simulink model "AutoPilot"  (R2013a)
settings: Solver=ode45  StartTime=0.0  StopTime=10.0  RelTol=1e-3
libraries: simulink x10
settings Model: Creator=falk  LastModifiedBy=falk

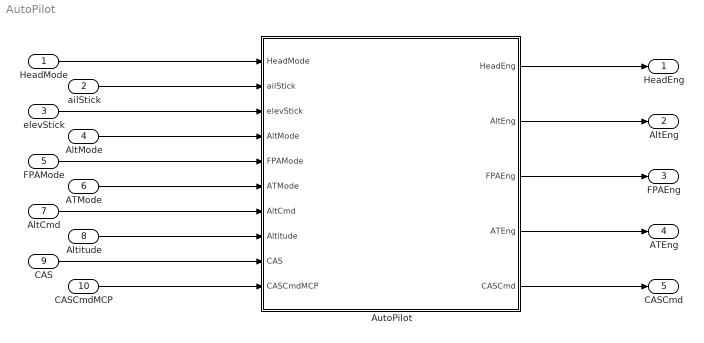
== system AutoPilot ==
  HeadMode : Inport
  ailStick : Inport  Port=2
  elevStick : Inport  Port=3
  AltMode : Inport  Port=4
  FPAMode : Inport  Port=5
  ATMode : Inport  Port=6
  AltCmd : Inport  Port=7
  Altitude : Inport  Port=8
  CAS : Inport  Port=9
  CASCmdMCP : Inport  Port=10
  AutoPilot : Subsystem
  HeadEng : Outport
  AltEng : Outport  Port=2
  FPAEng : Outport  Port=3
  ATEng : Outport  Port=4
  CASCmd : Outport  Port=5
  wires:
  HeadMode/1 -> AutoPilot/1(HeadMode)
  ailStick/1 -> AutoPilot/2(ailStick)
  elevStick/1 -> AutoPilot/3(elevStick)
  AltMode/1 -> AutoPilot/4(AltMode)
  FPAMode/1 -> AutoPilot/5(FPAMode)
  ATMode/1 -> AutoPilot/6(ATMode)
  AltCmd/1 -> AutoPilot/7(AltCmd)
  Altitude/1 -> AutoPilot/8(Altitude)
  CAS/1 -> AutoPilot/9(CAS)
  CASCmdMCP/1 -> AutoPilot/10(CASCmdMCP)
  AutoPilot/1(HeadEng) -> HeadEng/1
  AutoPilot/2(AltEng) -> AltEng/1
  AutoPilot/3(FPAEng) -> FPAEng/1
  AutoPilot/4(ATEng) -> ATEng/1
  AutoPilot/5(CASCmd) -> CASCmd/1

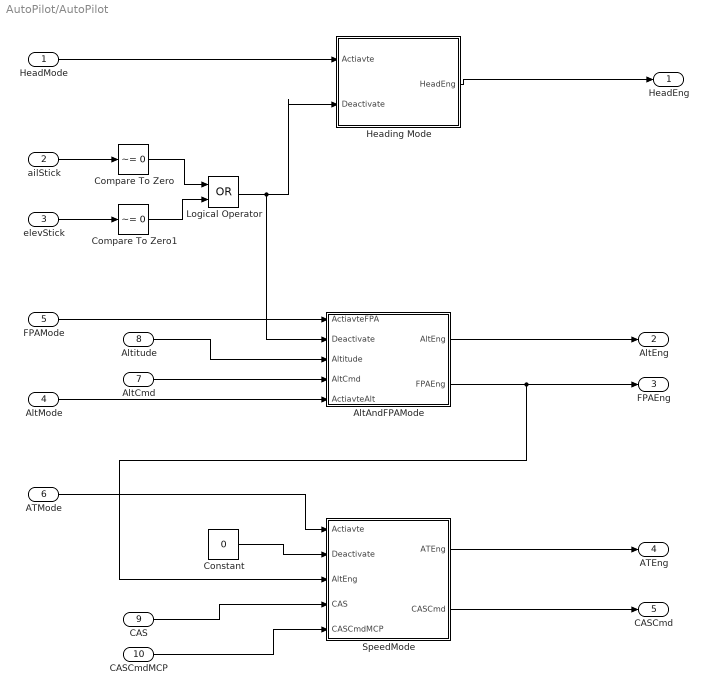
== system AutoPilot/AutoPilot ==
  HeadMode : Inport
  ailStick : Inport  Port=2
  elevStick : Inport  Port=3
  AltMode : Inport  Port=4
  FPAMode : Inport  Port=5
  ATMode : Inport  Port=6
  AltCmd : Inport  Port=7
  Altitude : Inport  Port=8
  CAS : Inport  Port=9
  CASCmdMCP : Inport  Port=10
  AltAndFPAMode : Subsystem
  Compare To Zero : simulink/Logic and Bit Operations/Compare To Zero  relop=~=  OutDataTypeStr=boolean
  Compare To Zero1 : simulink/Logic and Bit Operations/Compare To Zero  relop=~=  OutDataTypeStr=boolean
  Constant : Constant  Value=0
  Heading Mode : Subsystem
  Logical Operator : Logic  Operator=OR  AllPortsSameDT=off  OutDataTypeStr=boolean
  SpeedMode : Subsystem
  HeadEng : Outport
  AltEng : Outport  Port=2
  FPAEng : Outport  Port=3
  ATEng : Outport  Port=4
  CASCmd : Outport  Port=5
  wires:
  SpeedMode/1(ATEng) -> ATEng/1
  ailStick/1 -> Compare To Zero/1
  Constant/1 -> SpeedMode/2(Deactivate)
  AltAndFPAMode/2(FPAEng) -> FPAEng/1, SpeedMode/3(AltEng)
  AltAndFPAMode/1(AltEng) -> AltEng/1
  Heading Mode/1(HeadEng) -> HeadEng/1
  HeadMode/1 -> Heading Mode/1(Actiavte)
  Compare To Zero1/1 -> Logical Operator/2
  Compare To Zero/1 -> Logical Operator/1
  elevStick/1 -> Compare To Zero1/1
  ATMode/1 -> SpeedMode/1(Actiavte)
  FPAMode/1 -> AltAndFPAMode/1(ActiavteFPA)
  Altitude/1 -> AltAndFPAMode/3(Altitude)
  AltMode/1 -> AltAndFPAMode/5(ActiavteAlt)
  Logical Operator/1 -> AltAndFPAMode/2(Deactivate), Heading Mode/2(Deactivate)
  CASCmdMCP/1 -> SpeedMode/5(CASCmdMCP)
  AltCmd/1 -> AltAndFPAMode/4(AltCmd)
  SpeedMode/2(CASCmd) -> CASCmd/1
  CAS/1 -> SpeedMode/4(CAS)

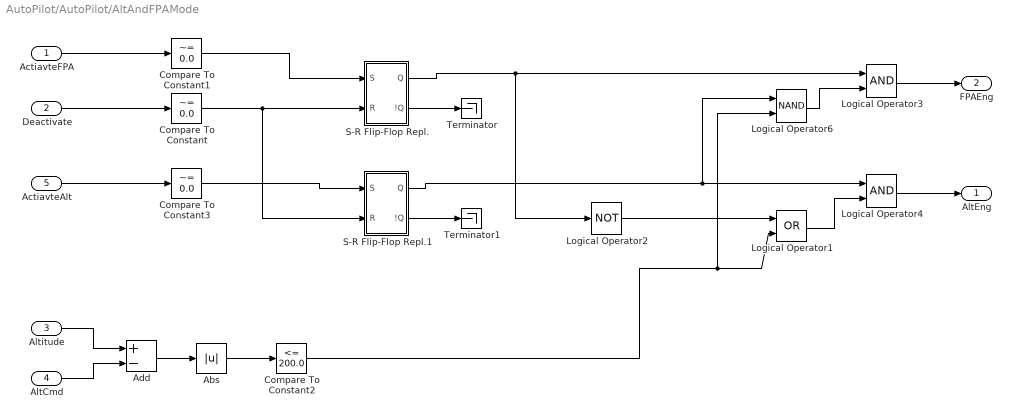
== system AutoPilot/AutoPilot/AltAndFPAMode ==
  ActiavteFPA : Inport
  Deactivate : Inport  Port=2
  Altitude : Inport  Port=3
  AltCmd : Inport  Port=4
  ActiavteAlt : Inport  Port=5
  Abs : Abs
  Add : Sum  Inputs=+-
  Compare To Constant : simulink/Logic and Bit Operations/Compare To Constant  relop=~=  const=0.0  OutDataTypeStr=boolean
  Compare To Constant1 : simulink/Logic and Bit Operations/Compare To Constant  relop=~=  const=0.0  OutDataTypeStr=boolean
  Compare To Constant2 : simulink/Logic and Bit Operations/Compare To Constant  relop=<=  const=200.0  OutDataTypeStr=boolean
  Compare To Constant3 : simulink/Logic and Bit Operations/Compare To Constant  relop=~=  const=0.0  OutDataTypeStr=boolean
  Logical Operator1 : Logic  Operator=OR  AllPortsSameDT=off  OutDataTypeStr=boolean
  Logical Operator2 : Logic  Operator=NOT  AllPortsSameDT=off  OutDataTypeStr=boolean
  Logical Operator3 : Logic  AllPortsSameDT=off  OutDataTypeStr=boolean
  Logical Operator4 : Logic  AllPortsSameDT=off  OutDataTypeStr=boolean
  Logical Operator6 : Logic  Operator=NAND  AllPortsSameDT=off  OutDataTypeStr=boolean
  S-R Flip-Flop Repl. : Subsystem
  S-R Flip-Flop Repl.1 : Subsystem
  Terminator : Terminator
  Terminator1 : Terminator
  AltEng : Outport
  FPAEng : Outport  Port=2
  wires:
  S-R Flip-Flop Repl./2(!Q) -> Terminator/1
  ActiavteFPA/1 -> Compare To Constant1/1
  S-R Flip-Flop Repl./1(Q) -> Logical Operator3/1, Logical Operator2/1
  Deactivate/1 -> Compare To Constant/1
  Compare To Constant1/1 -> S-R Flip-Flop Repl./1(S)
  S-R Flip-Flop Repl.1/2(!Q) -> Terminator1/1
  S-R Flip-Flop Repl.1/1(Q) -> Logical Operator6/1, Logical Operator4/1
  Compare To Constant3/1 -> S-R Flip-Flop Repl.1/1(S)
  Compare To Constant/1 -> S-R Flip-Flop Repl.1/2(R), S-R Flip-Flop Repl./2(R)
  ActiavteAlt/1 -> Compare To Constant3/1
  Altitude/1 -> Add/1
  AltCmd/1 -> Add/2
  Add/1 -> Abs/1
  Abs/1 -> Compare To Constant2/1
  Logical Operator3/1 -> FPAEng/1
  Logical Operator2/1 -> Logical Operator1/1
  Logical Operator4/1 -> AltEng/1
  Compare To Constant2/1 -> Logical Operator6/2, Logical Operator1/2
  Logical Operator1/1 -> Logical Operator4/2
  Logical Operator6/1 -> Logical Operator3/2

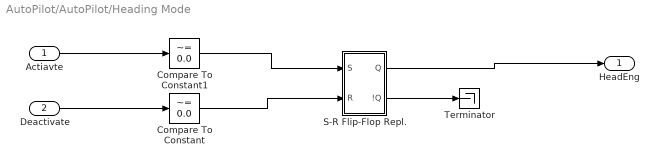
== system AutoPilot/AutoPilot/Heading Mode ==
  Actiavte : Inport
  Deactivate : Inport  Port=2
  Compare To Constant : simulink/Logic and Bit Operations/Compare To Constant  relop=~=  const=0.0  OutDataTypeStr=boolean
  Compare To Constant1 : simulink/Logic and Bit Operations/Compare To Constant  relop=~=  const=0.0  OutDataTypeStr=boolean
  S-R Flip-Flop Repl. : Subsystem
  Terminator : Terminator
  HeadEng : Outport
  wires:
  S-R Flip-Flop Repl./2(!Q) -> Terminator/1
  Actiavte/1 -> Compare To Constant1/1
  S-R Flip-Flop Repl./1(Q) -> HeadEng/1
  Deactivate/1 -> Compare To Constant/1
  Compare To Constant1/1 -> S-R Flip-Flop Repl./1(S)
  Compare To Constant/1 -> S-R Flip-Flop Repl./2(R)

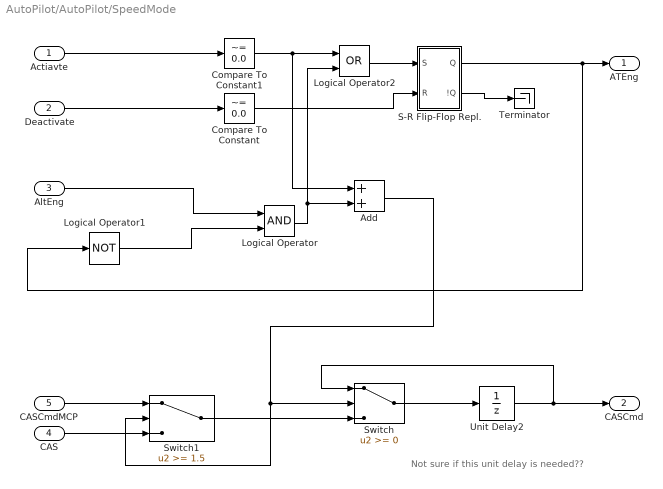
== system AutoPilot/AutoPilot/SpeedMode ==
  note: Not sure if this unit delay is needed??
  Actiavte : Inport
  Deactivate : Inport  Port=2
  AltEng : Inport  Port=3
  CAS : Inport  Port=4
  CASCmdMCP : Inport  Port=5
  Add : Sum
  Compare To Constant : simulink/Logic and Bit Operations/Compare To Constant  relop=~=  const=0.0  OutDataTypeStr=boolean
  Compare To Constant1 : simulink/Logic and Bit Operations/Compare To Constant  relop=~=  const=0.0  OutDataTypeStr=boolean
  Logical Operator : Logic  AllPortsSameDT=off  OutDataTypeStr=boolean
  Logical Operator1 : Logic  Operator=NOT  AllPortsSameDT=off  OutDataTypeStr=boolean
  Logical Operator2 : Logic  Operator=OR  AllPortsSameDT=off  OutDataTypeStr=boolean
  S-R Flip-Flop Repl. : Subsystem
  Switch : Switch
  Switch1 : Switch  Threshold=1.5
  Terminator : Terminator
  Unit Delay2 : UnitDelay  SampleTime=-1
  ATEng : Outport
  CASCmd : Outport  Port=2
  wires:
  S-R Flip-Flop Repl./2(!Q) -> Terminator/1
  Actiavte/1 -> Compare To Constant1/1
  S-R Flip-Flop Repl./1(Q) -> Logical Operator1/1, ATEng/1
  Deactivate/1 -> Compare To Constant/1
  Compare To Constant/1 -> S-R Flip-Flop Repl./2(R)
  AltEng/1 -> Logical Operator/1
  Logical Operator1/1 -> Logical Operator/2
  Logical Operator2/1 -> S-R Flip-Flop Repl./1(S)
  Logical Operator/1 -> Add/2, Logical Operator2/2
  CAS/1 -> Switch1/3
  CASCmdMCP/1 -> Switch1/1
  Compare To Constant1/1 -> Add/1, Logical Operator2/1
  Add/1 -> Switch1/2, Switch/2
  Switch1/1 -> Switch/3
  Switch/1 -> Unit Delay2/1
  Unit Delay2/1 -> Switch/1, CASCmd/1

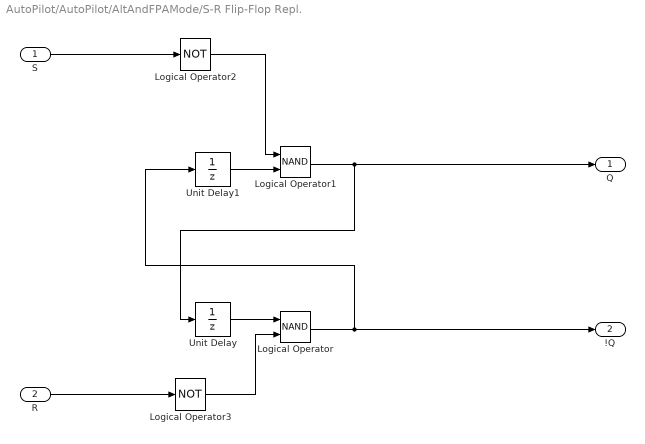
== system AutoPilot/AutoPilot/AltAndFPAMode/S-R Flip-Flop Repl. ==
  S : Inport
  R : Inport  Port=2
  Logical Operator : Logic  Operator=NAND  AllPortsSameDT=off  OutDataTypeStr=boolean
  Logical Operator1 : Logic  Operator=NAND  AllPortsSameDT=off  OutDataTypeStr=boolean
  Logical Operator2 : Logic  Operator=NOT  AllPortsSameDT=off  OutDataTypeStr=boolean
  Logical Operator3 : Logic  Operator=NOT  AllPortsSameDT=off  OutDataTypeStr=boolean
  Unit Delay : UnitDelay  SampleTime=-1
  Unit Delay1 : UnitDelay  InitialCondition=1  SampleTime=-1
  Q : Outport
  !Q : Outport  Port=2
  wires:
  Logical Operator/1 -> Unit Delay1/1, !Q/1
  Logical Operator1/1 -> Unit Delay/1, Q/1
  Unit Delay/1 -> Logical Operator/1
  Unit Delay1/1 -> Logical Operator1/2
  Logical Operator2/1 -> Logical Operator1/1
  Logical Operator3/1 -> Logical Operator/2
  R/1 -> Logical Operator3/1
  S/1 -> Logical Operator2/1

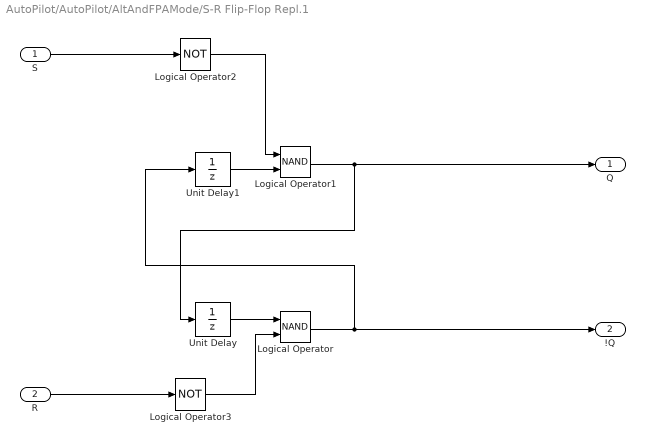
== system AutoPilot/AutoPilot/AltAndFPAMode/S-R Flip-Flop Repl.1 ==
  S : Inport
  R : Inport  Port=2
  Logical Operator : Logic  Operator=NAND  AllPortsSameDT=off  OutDataTypeStr=boolean
  Logical Operator1 : Logic  Operator=NAND  AllPortsSameDT=off  OutDataTypeStr=boolean
  Logical Operator2 : Logic  Operator=NOT  AllPortsSameDT=off  OutDataTypeStr=boolean
  Logical Operator3 : Logic  Operator=NOT  AllPortsSameDT=off  OutDataTypeStr=boolean
  Unit Delay : UnitDelay  SampleTime=-1
  Unit Delay1 : UnitDelay  InitialCondition=1  SampleTime=-1
  Q : Outport
  !Q : Outport  Port=2
  wires:
  Logical Operator/1 -> Unit Delay1/1, !Q/1
  Logical Operator1/1 -> Unit Delay/1, Q/1
  Unit Delay/1 -> Logical Operator/1
  Unit Delay1/1 -> Logical Operator1/2
  Logical Operator2/1 -> Logical Operator1/1
  Logical Operator3/1 -> Logical Operator/2
  R/1 -> Logical Operator3/1
  S/1 -> Logical Operator2/1

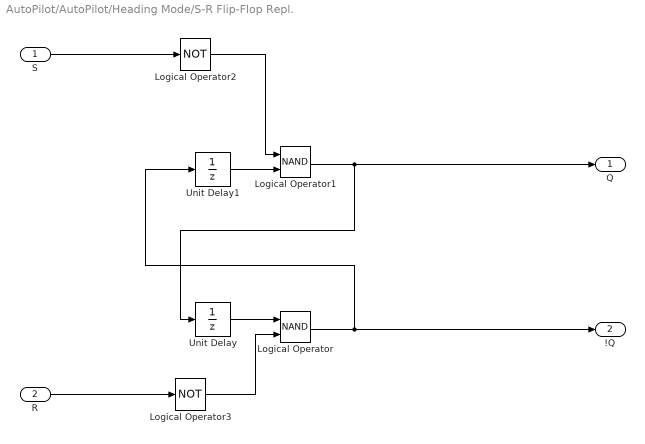
== system AutoPilot/AutoPilot/Heading Mode/S-R Flip-Flop Repl. ==
  S : Inport
  R : Inport  Port=2
  Logical Operator : Logic  Operator=NAND  AllPortsSameDT=off  OutDataTypeStr=boolean
  Logical Operator1 : Logic  Operator=NAND  AllPortsSameDT=off  OutDataTypeStr=boolean
  Logical Operator2 : Logic  Operator=NOT  AllPortsSameDT=off  OutDataTypeStr=boolean
  Logical Operator3 : Logic  Operator=NOT  AllPortsSameDT=off  OutDataTypeStr=boolean
  Unit Delay : UnitDelay  SampleTime=-1
  Unit Delay1 : UnitDelay  InitialCondition=1  SampleTime=-1
  Q : Outport
  !Q : Outport  Port=2
  wires:
  Logical Operator/1 -> Unit Delay1/1, !Q/1
  Logical Operator1/1 -> Unit Delay/1, Q/1
  Unit Delay/1 -> Logical Operator/1
  Unit Delay1/1 -> Logical Operator1/2
  Logical Operator2/1 -> Logical Operator1/1
  Logical Operator3/1 -> Logical Operator/2
  R/1 -> Logical Operator3/1
  S/1 -> Logical Operator2/1

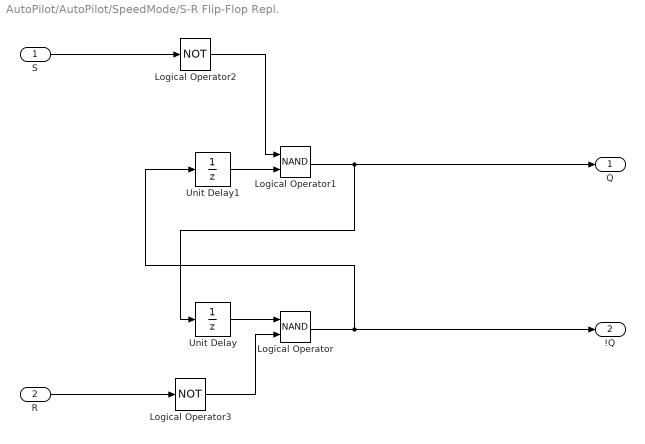
== system AutoPilot/AutoPilot/SpeedMode/S-R Flip-Flop Repl. ==
  S : Inport
  R : Inport  Port=2
  Logical Operator : Logic  Operator=NAND  AllPortsSameDT=off  OutDataTypeStr=boolean
  Logical Operator1 : Logic  Operator=NAND  AllPortsSameDT=off  OutDataTypeStr=boolean
  Logical Operator2 : Logic  Operator=NOT  AllPortsSameDT=off  OutDataTypeStr=boolean
  Logical Operator3 : Logic  Operator=NOT  AllPortsSameDT=off  OutDataTypeStr=boolean
  Unit Delay : UnitDelay  SampleTime=-1
  Unit Delay1 : UnitDelay  InitialCondition=1  SampleTime=-1
  Q : Outport
  !Q : Outport  Port=2
  wires:
  Logical Operator/1 -> Unit Delay1/1, !Q/1
  Logical Operator1/1 -> Unit Delay/1, Q/1
  Unit Delay/1 -> Logical Operator/1
  Unit Delay1/1 -> Logical Operator1/2
  Logical Operator2/1 -> Logical Operator1/1
  Logical Operator3/1 -> Logical Operator/2
  R/1 -> Logical Operator3/1
  S/1 -> Logical Operator2/1
